simulink model "SSMC_Ate"  (R2026b)
settings Model: Creator=Yahoff  LastModifiedBy=Yahoff

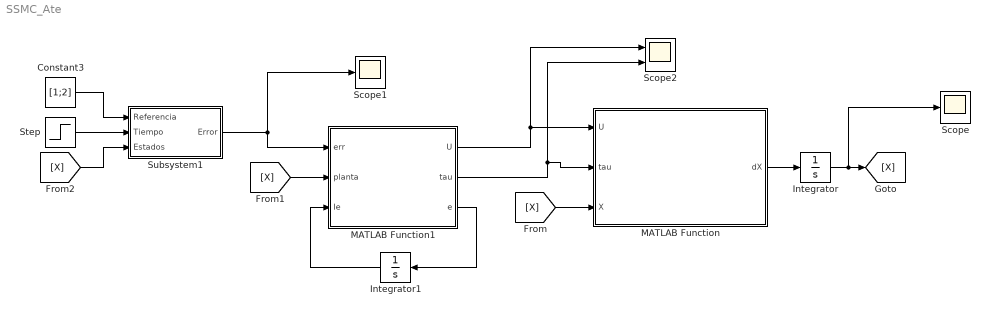
== system SSMC_Ate ==
  Constant3 : Constant  Value=[1;2]
  Integrator : Integrator  InitialCondition=[0;0;0;0;0;0]
  Integrator1 : Integrator
  MATLAB Function : MATLAB Function  TreatAsAtomicUnit=on
  MATLAB Function1 : MATLAB Function  TreatAsAtomicUnit=on
  Scope : Scope
      settings: ActiveDisplayYMinimum=-0.2512466571019662  ActiveDisplayYMaximum=2.2612199139176963
  Scope1 : Scope
      settings: ActiveDisplayYMinimum=-0.26245750143574675  ActiveDisplayYMaximum=0.2179150564198867
  Scope2 : Scope  NumInputPorts=2
      settings: ActiveDisplayYMinimum=7.3180451713334094  ActiveDisplayYMaximum=20.198683924690176  DataLoggingVariableName=ScopeData2
  Step : Step  SampleTime=0
  Subsystem1 : Subsystem
  wires:
  MATLAB Function/1(dX) -> Integrator/1
  Integrator/1 -> Scope/1, [X]
  [X] -> MATLAB Function/3(X)
  [X] -> MATLAB Function1/2(planta)
  [X] -> Subsystem1/3(Estados)
  Constant3/1 -> Subsystem1/1(Referencia)
  Subsystem1/1(Error) -> Scope1/1, MATLAB Function1/1(err)
  MATLAB Function1/2(tau) -> Scope2/2, MATLAB Function/2(tau)
  MATLAB Function1/1(U) -> Scope2/1, MATLAB Function/1(U)
  Integrator1/1 -> MATLAB Function1/3(Ie)
  MATLAB Function1/3(e) -> Integrator1/1
  Step/1 -> Subsystem1/2(Tiempo)

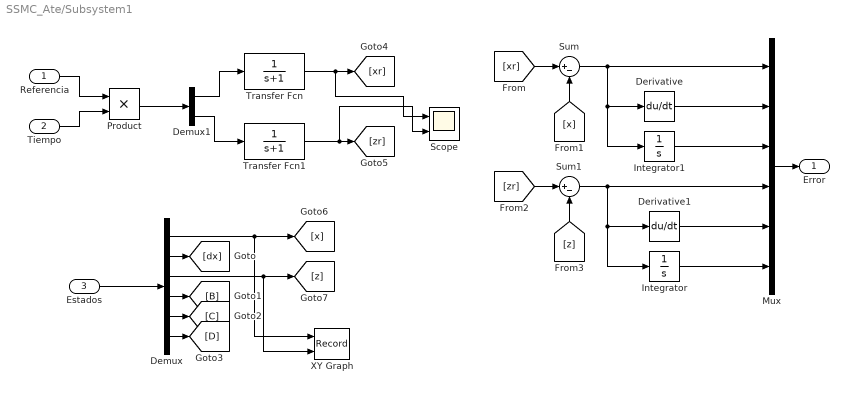
== system SSMC_Ate/Subsystem1 ==
  Referencia : Inport
  Tiempo : Inport  Port=2
  Estados : Inport  Port=3
  Demux : Demux  Outputs=6
  Demux1 : Demux  Outputs=2
  Derivative : Derivative
  Derivative1 : Derivative
  Integrator : Integrator
  Integrator1 : Integrator
  Mux : Mux  Inputs=6
  Product : Product
  Scope : Scope  NumInputPorts=2
      settings: ActiveDisplayYMinimum=-0.24996915269105333  ActiveDisplayYMaximum=2.2497223742194805  DataLoggingVariableName=ScopeData3
  Sum : Sum  Inputs=|+-
  Sum1 : Sum  Inputs=|+-
  Transfer Fcn : TransferFcn  Denominator=[1 1]
  Transfer Fcn1 : TransferFcn  Denominator=[1 1]
  XY Graph : Record  NumPorts=2.0  FileSettingsInternal="{\"entries\":[{\"content\":{\"excelSettings\":{\"content\":{},\"type\":\"Streamout.ExcelSettings\"},\"parquetSettings\":{\"content\":{},\"type\":\"Streamout.ParquetSettings\"}},\"type\":\"Streamout.FileSettingStorage\",\"uuid\":\"\"}],\"packageUris\":[\"http:\\/\\/schema.mathworks.com\\/mf0\\/streamout_blocks\\/R2020a\"],\"version\":\"1.0\"}"  FrameSettings=[0, 0]  Layout=[1 1]  SignalsInternal="{\"entries\":[{\"content\":{\"signals\":[{\"content\":{\"blockPath\":[],\"dimensions\":[1],\"domain\":\"\",\"lineColor\":\"#a2142f\",\"plots\":[ 1 ],\"port\":1,\"sid\":[\"\"],\"signalID\":1,\"signalName\":\"Demux:1\"},\"type\":\"RecordBlkView.Signal\",\"uuid\":\"\"},{\"content\":{\"blockPath\":[],\"dimensions\":[1],\"domain\":\"\",\"lineColor\":\"#139fff\",\"plots\":[ 1 ],\"port\":2,\"sid\":[\"\"],\"signalID\":2,\"signalName\":\"Demux:3\"},\"type\":\"RecordBlkView.Signal\",\"uuid\":\"\"}]},\"type\":\"RecordBlkView.InputSignals\",\"uuid\":\"\"}],\"packageUris\":[\"http:\\/\\/schema.mathworks.com\\/mf0\\/streamout_blocks\\/R2020a\"],\"version\":\"1.0\"}"  VisualizationBindings="{\"xyplotplugin\":{\"info\":[{\"series\":[{\"bindingParametersList\":[{\"parameter\":\"X-Axis\",\"signalID\":1,\"signalName\":\"Demux:1\"},{\"parameter\":\"Y-Axis\",\"signalID\":2,\"signalName\":\"Demux:3\"}],\"seriesID\":0}],\"subplotID\":1}]}}"  CompatibilityTag=XY
  Error : Outport
  wires:
  Demux/3 -> XY Graph/2, [z]
  Demux/1 -> XY Graph/1, [x]
  Demux/5 -> [C]
  Demux/6 -> [D]
  Estados/1 -> Demux/1
  Demux/2 -> [dx]
  Demux/4 -> [B]
  Referencia/1 -> Product/1
  Tiempo/1 -> Product/2
  Product/1 -> Demux1/1
  Demux1/2 -> Transfer Fcn1/1
  Demux1/1 -> Transfer Fcn/1
  Transfer Fcn/1 -> Scope/1, [xr]
  Transfer Fcn1/1 -> Scope/2, [zr]
  [xr] -> Sum/1
  [x] -> Sum/2
  [zr] -> Sum1/1
  [z] -> Sum1/2
  Sum/1 -> Integrator1/1, Derivative/1, Mux/1
  Sum1/1 -> Integrator/1, Derivative1/1, Mux/4
  Derivative/1 -> Mux/2
  Mux/1 -> Error/1
  Derivative1/1 -> Mux/5
  Integrator/1 -> Mux/6
  Integrator1/1 -> Mux/3

== matlab function SSMC_Ate/MATLAB Function1 ==
  data: err input; U output; planta input; tau output; Ie input; e output
function [U, tau,e] = control(err, planta,Ie)

    m = 1; g = 9.81;
    kth = 100; kom =50;

    k=4;%4
    m=1;%1
    l=1;%2
    n=1;%1

    ex  = err(1);
    dex = err(2);
    Iex = err(3);   
    ez  = err(4);
    dez = err(5);
    Iez = err(6);

    x     = planta(1);
    dx    = planta(2);
    z     = planta(3);
    dz  = planta(4);
    th    = planta(5);
    thdot = planta(6);

    Vex = l + n*abs(dx) + n*abs(ex);
    s   = dex + n*ex + n*Iex;
    vx  = k*Vex*sat(s);
   
    Vez = l + n*abs(dz) + n*abs(ez);
    s   = dez + n*ez + n*Iez;
    vz  = k*Vez*sat(s);

    U   = m*sqrt(vx^2 + (vz+g)^2);
    thd = atan2(-vx, vz+g);

    e = th - thd;
    de = thdot;

    Ka = 3;
    La = 100;
    na = 10;

    Vet = -La + na*abs(de) + na*abs(e);
    st   = de + na*e + na*Ie;
    tau  = + Ka*Vet*sign(st);
end



function y = sat(u)
if u > 1
    y = 1;
elseif u < -1
    y = -1;
else
    y = u;
end
end

== matlab function SSMC_Ate/MATLAB Function ==
  data: U input; dX output; tau input; X input
function dX = planta(U, tau, X)

    m = 1; J = 1; g = 9.81;
    kth = 30; kom = 12;

    x     = X(1);
    xdot  = X(2);
    z     = X(3);
    zdot  = X(4);
    th    = X(5);
    thdot = X(6);

    xdd  = -(U/m)*sin(th);
    zdd  =  (U/m)*cos(th) - g;
    thdd =  tau/J;

    dX = [xdot; xdd; zdot; zdd; thdot; thdd];
